simulink model "ARX_simu_DS"  (R2022b)
settings: Solver=ode4  StartTime=Ts  StopTime=T  FixedStep=Ts  RelTol=1e-3  EnableMultiTasking=on
values from neighbouring files (symbols this model uses):
  A1 = 2 * a * r1 - a    [GWO_PID_Update.m]
  A2 = 2 * a * r1 - a    [GWO_PID_Update.m]
  C1 = 2 * r2    [GWO_PID_Update.m]
  C2 = 2 * r2    [GWO_PID_Update.m]
  Ts = 1 + S    [BE_discretize_PID.m]    (also in Strategie_Cautare.m = 1)
  y1_ref = Y_ref(1,1)    [Functia_Fitness_AM_Noua.m]    (also in Strategie_Cautare.m = Y_ref(:,1))
  y2_ref = Y_ref(1,2)    [Functia_Fitness_AM_Noua.m]    (also in Strategie_Cautare.m = Y_ref(:,2))
undefined symbols (not defined in the file or in its folder): ARX1_ini, ARX2_ini, B11, B12, B21, B22, D1, D2, R11, R12, R21, R22, S11, S12, S21, S22, U_max, U_min, Y_max, Y_min
libraries: simulink x2
settings Model: ModifiedComment=Administrator -- Tue Mar 09 18:29:07 2021 -- Version 1.295  Creator=Razvan  LastModifiedBy=Asus
settings Model: ModifiedHistory=|
  | Administrator -- Tue Mar 09 18:29:07 2021 -- Version 1.295
  | 
  | Administrator -- Tue Mar 09 18:11:42 2021 -- Version 1.294
settings SolverCC: AlgebraicLoopSolver=TrustRegion
settings DataIOCC: ExternalInput=[t, ref1,ref2]  SaveOutput=off  SaveTime=off  ReturnWorkspaceOutputs=off
settings OptimizationCC: LifeSpan=inf
settings DebuggingCC: UnconnectedInputMsg=warning  UnconnectedOutputMsg=warning  UnconnectedLineMsg=warning  SFUnexpectedBacktrackingDiag=warning  SFNoUnconditionalDefaultTransitionDiag=warning  SFExecutionAtInitializationDiag=none  SFMachineParentedDataDiag=warning  ArithmeticOperatorsInVariantConditions=warning
settings ModelReferenceCC: EnableRefExpFcnMdlSchedulingChecks=on
settings SFSimCC: SimUseLocalCustomCode=off  CustomCodeUndefinedFunction=UseInterfaceOnly
settings RTWCC: RTWUseLocalCustomCode=off
settings CodeAppCC: StateflowObjectComments=on
settings GRTTargetCC: TargetLangStandard=C89/C90 (ANSI)
settings ConfigComp: CovMetricSettings=dw  CovSaveCumulativeToWorkspaceVar=on  CovSaveSingleToWorkspaceVar=on  CovExternalEMLEnable=off

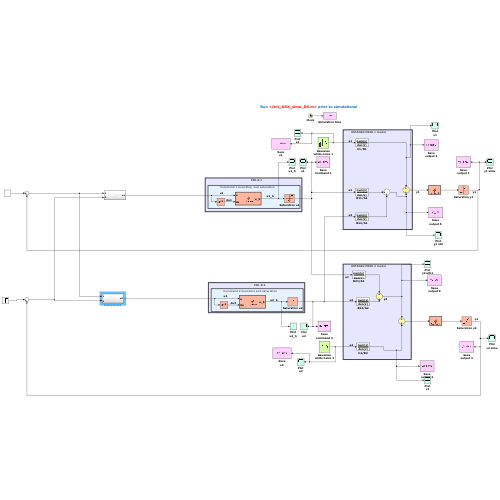
[thumbnail: Simulink's stored preview of the top-level diagram]
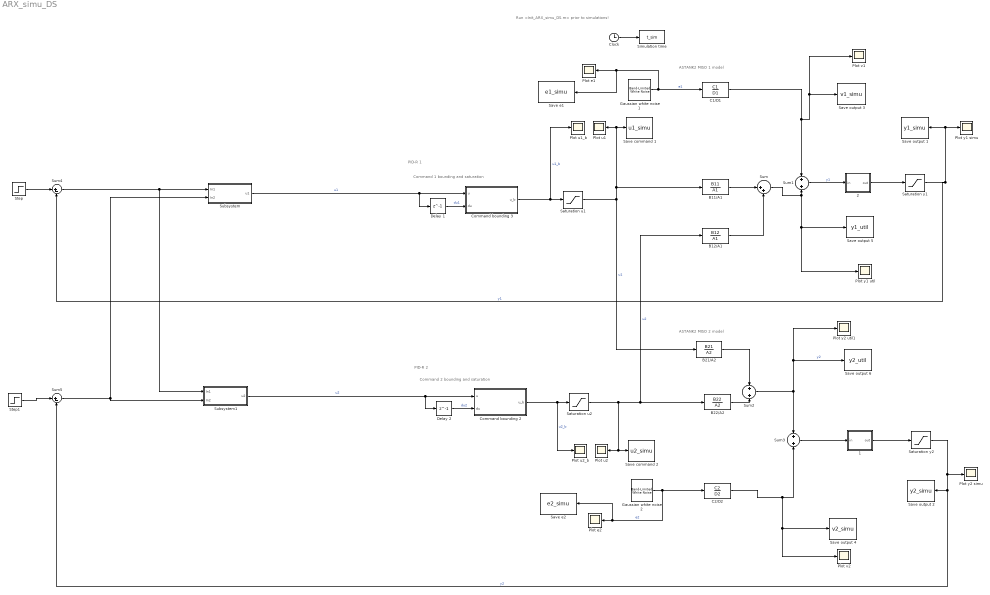
== system ARX_simu_DS ==
  note: PID-R 1
  note: PID-R 2
  note: ASTANK2 MISO 1 model
  note: Command 1 bounding and saturation
  note: Run <Init_ARX_simu_DS.m> prior to simulations!
  note: ASTANK2 MISO 2 model
  note: Command 2 bounding and saturation
  " 1" : MATLAB Function  TreatAsAtomicUnit=on
  " 2" : MATLAB Function  TreatAsAtomicUnit=on
  B11/A1 : DiscreteFilter  Numerator=B11  Denominator=A1  InitialStates=ARX1_ini.b1  SampleTime=Ts
  B12/A1 : DiscreteFilter  Numerator=B12  Denominator=A1  InitialStates=ARX1_ini.b2  SampleTime=Ts
  B21/A2 : DiscreteFilter  Numerator=B21  Denominator=A2  InitialStates=ARX2_ini.b1  SampleTime=Ts
  B22/A2 : DiscreteFilter  Numerator=B22  Denominator=A2  InitialStates=ARX2_ini.b2  SampleTime=Ts
  C1/D1 : DiscreteFilter  Numerator=C1  Denominator=D1  SampleTime=Ts
  C2/D2 : DiscreteFilter  Numerator=C2  Denominator=D2  SampleTime=Ts
  Clock : Clock
  Command bounding 2 : MATLAB Function  TreatAsAtomicUnit=on
  Command bounding 3 : MATLAB Function  TreatAsAtomicUnit=on
  Delay 1 : Delay  DelayLength=1
  Delay 2 : Delay  DelayLength=1
  Gaussian white noise 1 : simulink/Sources/Band-Limited White Noise  Cov=lambda12  Ts=Ts  seed=seed1
  Gaussian white noise 2 : simulink/Sources/Band-Limited White Noise  Cov=lambda22  Ts=Ts  seed=seed2
  Plot e1 : Scope
  Plot e2 : Scope
  Plot u1 : Scope
  Plot u1_b : Scope
  Plot u2 : Scope
  Plot u2_b : Scope
  Plot v1 : Scope
  Plot v2 : Scope
  Plot y1 simu : Scope
  Plot y1 util : Scope
  Plot y2 simu : Scope
  Plot y2 util1 : Scope
  Saturation u1 : Saturate  UpperLimit=U_max  LowerLimit=U_min
  Saturation u2 : Saturate  UpperLimit=U_max  LowerLimit=U_min
  Saturation y1 : Saturate  UpperLimit=Y_max  LowerLimit=Y_min
  Saturation y2 : Saturate  UpperLimit=Y_max  LowerLimit=Y_min
  Save command 1 : ToWorkspace  VariableName=u1_simu  SampleTime=Ts
  Save command 2 : ToWorkspace  VariableName=u2_simu  SampleTime=Ts
  Save e1 : ToWorkspace  VariableName=e1_simu  SampleTime=Ts
  Save e2 : ToWorkspace  VariableName=e2_simu  SampleTime=Ts
  Save output 1 : ToWorkspace  VariableName=y1_simu  SampleTime=Ts
  Save output 2 : ToWorkspace  VariableName=y2_simu  SampleTime=Ts
  Save output 3 : ToWorkspace  VariableName=v1_simu  SampleTime=Ts
  Save output 4 : ToWorkspace  VariableName=v2_simu  SampleTime=Ts
  Save output 5 : ToWorkspace  VariableName=y1_util  SampleTime=Ts
  Save output 6 : ToWorkspace  VariableName=y2_util  SampleTime=Ts
  Simulation time : ToWorkspace  VariableName=t_sim  SampleTime=Ts
  Step : Step  Time=0  After=y1_ref  SampleTime=Ts
  Step1 : Step  Time=0  After=y2_ref  SampleTime=Ts
  Subsystem : Subsystem  Description=PID-1
  Subsystem1 : Subsystem
  Sum : Sum  Inputs=|++
  Sum1 : Sum
  Sum2 : Sum
  Sum3 : Sum
  Sum4 : Sum  Inputs=|+-
  Sum5 : Sum  Inputs=|+-
  wires:
  Sum1/1 -> " 2"/1(in)  "y1"
  Saturation u1/1 -> B21/A2/1, B11/A1/1, Save command 1/1, Plot u1/1  "u1"
  Subsystem/1(u1) -> Delay 1/1, Command bounding 3/1(u)  "u1"
  Command bounding 3/1(u_b) -> Plot u1_b/1, Saturation u1/1  "u1_b"
  Delay 1/1 -> Command bounding 3/2(du)  "du1"
  Clock/1 -> Simulation time/1
  B11/A1/1 -> Sum/1
  C1/D1/1 -> Sum1/1, Plot v1/1, Save output 3/1
  Gaussian white noise 1/1 -> C1/D1/1, Save e1/1, Plot e1/1  "e1"
  Delay 2/1 -> Command bounding 2/2(du)  "du2"
  Command bounding 2/1(u_b) -> Plot u2_b/1, Saturation u2/1  "u2_b"
  Saturation u2/1 -> B22/A2/1, B12/A1/1, Save command 2/1, Plot u2/1  "u2"
  Subsystem1/1(u2) -> Delay 2/1, Command bounding 2/1(u)  "u2"
  B22/A2/1 -> Sum2/2
  Gaussian white noise 2/1 -> C2/D2/1, Save e2/1, Plot e2/1  "e2"
  B21/A2/1 -> Sum2/1
  " 2"/1(out) -> Saturation y1/1
  " 1"/1(out) -> Saturation y2/1
  Saturation y1/1 -> Sum4/2, Save output 1/1, Plot y1 simu/1  "y1"
  Saturation y2/1 -> Sum5/2, Save output 2/1, Plot y2 simu/1  "y2"
  B12/A1/1 -> Sum/2
  Sum/1 -> Plot y1 util/1, Save output 5/1, Sum1/2
  Sum2/1 -> Sum3/1, Plot y2 util1/1, Save output 6/1  "y2"
  C2/D2/1 -> Plot v2/1, Save output 4/1, Sum3/2
  Sum3/1 -> " 1"/1(in)
  Step1/1 -> Sum5/1
  Step/1 -> Sum4/1
  Sum4/1 -> Subsystem1/1(In1), Subsystem/1(In1)
  Sum5/1 -> Subsystem1/2(In2), Subsystem/2(In2)

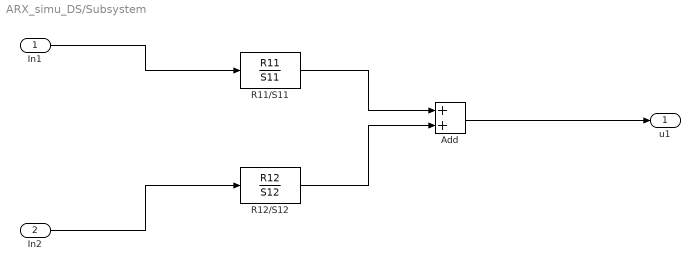
== system ARX_simu_DS/Subsystem ==
  In1 : Inport
  In2 : Inport  Port=2
  Add : Sum
  R11/S11 : DiscreteFilter  Numerator=R11  Denominator=S11
  R12/S12 : DiscreteFilter  Numerator=R12  Denominator=S12
  u1 : Outport  Tag=u2
  wires:
  In1/1 -> R11/S11/1
  In2/1 -> R12/S12/1
  R11/S11/1 -> Add/1
  R12/S12/1 -> Add/2
  Add/1 -> u1/1

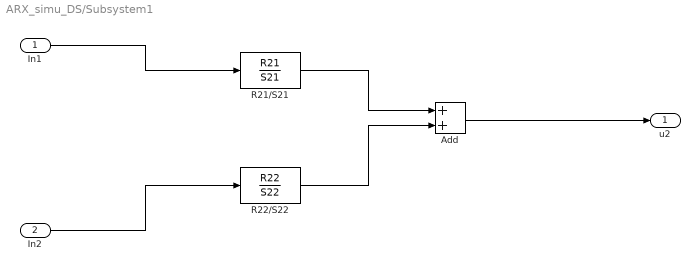
== system ARX_simu_DS/Subsystem1 ==
  In1 : Inport
  In2 : Inport  Port=2
  Add : Sum
  R21/S21 : DiscreteFilter  Numerator=R21  Denominator=S21
  R22/S22 : DiscreteFilter  Numerator=R22  Denominator=S22
  u2 : Outport
  wires:
  In1/1 -> R21/S21/1
  In2/1 -> R22/S22/1
  R21/S21/1 -> Add/1
  R22/S22/1 -> Add/2
  Add/1 -> u2/1

== matlab function ARX_simu_DS/Command bounding 3 ==
  data: u input; du input; u_b output
function u_b = u_bound(u,du)

u_b = max(du-3,min(du+3,u)) ;

== matlab function ARX_simu_DS/ 1 ==
  data: in input; out output
function out = NaN2null(in)

if (isnan(in))
    out = 0 ; 
else
    out = in ;
end ;

== matlab function ARX_simu_DS/ 2 ==
  data: in input; out output
function out = NaN2null(in)

if (isnan(in))
    out = 0 ; 
else
    out = in ;
end ;

== matlab function ARX_simu_DS/Command bounding 2 ==
  data: u input; du input; u_b output
function u_b = u_bound(u,du)

u_b = max(du-3,min(du+3,u)) ;
